simulink model "practica2b"  (R2022a)
settings: Solver=FixedStepAuto  StartTime=0.0  StopTime=10.0  RelTol=1e-3  EnableMultiTasking=on
undefined symbols (not defined in the file): ni, ref, t_sim
libraries: legoev3lib x6, simulink x1
settings Model: ExtModeTrigDuration=2  Creator=alumnopr09  LastModifiedBy=Sersa
settings SolverCC: AlgebraicLoopSolver=TrustRegion  PositivePriorityOrder=on
settings OptimizationCC: EnhancedBackFolding=on  PassReuseOutputArgsAs=Individual arguments  ZeroExternalMemoryAtStartup=off  ZeroInternalMemoryAtStartup=off  MaxStackSize=64  OptimizeBlockOrder=speed  DifferentSizesBufferReuse=on  OptimizationCustomize=off  EfficientTunableParamExpr=on
settings DebuggingCC: ParameterTunabilityLossMsg=error  UnconnectedInputMsg=warning  UnconnectedOutputMsg=warning  UnconnectedLineMsg=warning  SFMachineParentedDataDiag=warning
settings HardwareCC: ProdBitPerPointer=32  ProdBitPerSizeT=32  ProdBitPerPtrDiffT=32  ProdLargestAtomicInteger=Long  ProdWordSize=32  ProdHWDeviceType=ARM Compatible->ARM 9
settings SFSimCC: MATLABDynamicMemAlloc=off
settings RTWCC: SystemTargetFile=ert.tlc  HardwareBoard=LEGO MINDSTORMS EV3  TLCOptions="-aInlineSetEventsForThisBaseRateFcn=TLC_FALSE -aSuppressMultiTaskScheduler=TLC_FALSE  -aRateBasedStepFcn=0"  TemplateMakefile=ert_default_tmf  GenerateReport=on  Toolchain=Sourcery G++ Lite v2009q3  IncludeHyperlinkInReport=on  LaunchReport=on  GenerateTraceInfo=on  GenerateTraceReport=on  GenerateTraceReportSl=on  GenerateTraceReportSf=on  GenerateTraceReportEml=on
settings CodeAppCC: ForceParamTrailComments=on  IgnoreCustomStorageClasses=off  OperatorAnnotations=on  SimulinkDataObjDesc=on  SFDataObjDesc=on  InsertBlockDesc=on
settings ERTTargetCC: SupportContinuousTime=on  SupportVariableSizeSignals=on

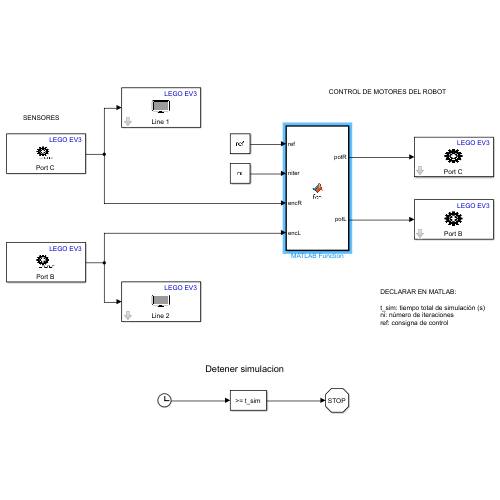
[thumbnail: Simulink's stored preview of the top-level diagram]
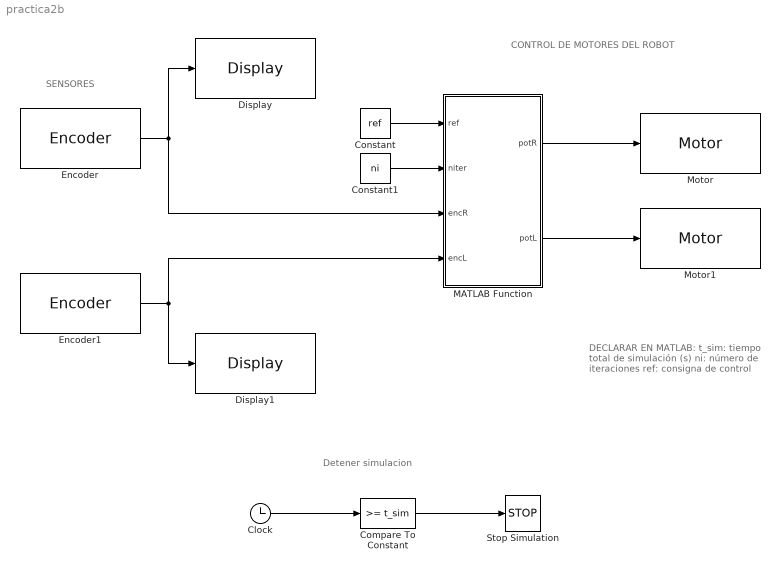
== system practica2b ==
  note: DECLARAR EN MATLAB:
      |
      | t_sim: tiempo total de simulación (s)
      | ni: número de iteraciones
      | ref: consigna de control
  note: CONTROL DE MOTORES DEL ROBOT
  note: SENSORES
  note: Detener simulacion
  Clock : Clock
  Compare To Constant : simulink/Logic and Bit Operations/Compare To Constant  relop=>=  const=t_sim  OutDataTypeStr=boolean
  Constant : Constant  Value=ref
  Constant1 : Constant  Value=ni
  Display : legoev3lib/Display  slcdLine=1  slcdFormat=Decimal
      settings: SourceProductBaseCode=LEGOEV3
  Display1 : legoev3lib/Display  slcdLine=2  slcdFormat=Decimal
      settings: SourceProductBaseCode=LEGOEV3
  Encoder : legoev3lib/Encoder  portNumber=C  opMode=No reset  sampleTime=0.1
      settings: SourceProductBaseCode=LEGOEV3
  Encoder1 : legoev3lib/Encoder  portNumber=B  opMode=No reset  sampleTime=0.1
      settings: SourceProductBaseCode=LEGOEV3
  MATLAB Function : MATLAB Function  TreatAsAtomicUnit=on
  Motor : legoev3lib/Motor  sportNumber=C  sstopAction=Brake
  Motor1 : legoev3lib/Motor  sportNumber=B  sstopAction=Brake
  Stop Simulation : Stop
  wires:
  Clock/1 -> Compare To Constant/1
  Compare To Constant/1 -> Stop Simulation/1
  Encoder/1 -> MATLAB Function/3(encR), Display/1
  Encoder1/1 -> MATLAB Function/4(encL), Display1/1
  MATLAB Function/1(potR) -> Motor/1
  MATLAB Function/2(potL) -> Motor1/1
  Constant1/1 -> MATLAB Function/2(niter)
  Constant/1 -> MATLAB Function/1(ref)

== matlab function practica2b/MATLAB Function ==
  data: ref input; potR output; niter input; encR input; encL input; potL output
function [potR,potL]    = fcn(ref,niter,encR,encL)
    persistent iter;
    
    if (isempty(iter))
        iter = 0;
    end
    
    iter = iter +1;
    
    if(iter <= niter)
        potR = int32(ref-encR);
        potL = int32(ref-encL);
        
        if(potR>100)
            potR=int32(100);
        elseif(potR<-100)
            potR = int32(-100);
        end
        
        if(potL>100)
            potL=int32(100);
        elseif(potL<-100)
            potL = int32(-100);
        end
        
    else
        potR =int32(0);
        potL =int32(0);
    end
